simulink model "ML_2L_GFL_Y_Measure_AC_Sweep_2023"  (R2021b)
settings: Solver=ode23tb  StartTime=0.0  StopTime=1  FixedStep=Ts_Power  RelTol=1e-5
PreLoadFcn:
  | %Ts_Power=10e-6;
  | %Ts_Control=50e-6;
  | % System parameters
  | %Vl_l  = 400;   			        % Grid line-to-line voltage (Vrms)
  | %Vg_peak = Vl_l/sqrt(3)*sqrt(2); % Grid phase voltage (Vpk)
  | fg     = 50;	  			        % grid frequency (Hz)
  | %P = 30e3;
  | %Q = 0;
  | % LCL Filter parameters
  | L1=3e-3;
  | R_L1=80e-3;
  | L2=1.7e-3;
  | R_L2=22.3e-3;
  | C1=2e-6;
  | R_C1=7+21.5e-3;
  | % DC-link parameters
  | Vdc = 700;             	% DC voltage (V)
  | C=1500e-6;					% DC-link capacitance (F)
  | ESP=1e-3;
  | % Control parameters
  | fs = 10e3; 					% Switching frequency (Hz)
  | ts = 1/fs; 					% Switching period (s)
  | % Device parameters
  | Ron=1e-3;
  | 
  | 
  | 
  | % Circuit parameters
  | %Pr = 10000;            % Rated power (W)
  | %Zb = Vg_rms^2/Pr;     	% Base impedance (Ohm)
  | %Lg = 0.1*Zb/(2*pi*fac);% Grid connecting reactance (H)
  | %Rg = 0.01*Zb;         	% Grid connecting resistance (Ohm)
  | 
  | % Determining initial conditions
  | %Zinv = Rg + 1i*2*pi*fac*Lg;% Connecting impedance (Ohm,complex)
  | %Iref = Pr/(3*Vg_rms);      % Reference current (Irms)
  | %Vinv = Vg_rms + Iref*Zinv; % VSI generated voltage (Vrms,complex)
  | %Vinv_rms = abs(Vinv);      % VSI generated voltage magnitude (Vrms)
  | %Vinv_angle= angle(Vinv);   % VSI generated voltage angle (Rads)
  | 
  | %phase_balanced = 2*pi/3*[0 -1 1]; % Ideal balanced three-phase angles (Rads)
  | 
  | % Sine and Space Vector PWM parameters
  | %Vref = Vinv_rms*sqrt(2);  	% Reference voltage amplitude (V)
  | %phase_sine  = phase_balanced + Vinv_angle;   % Angles for sine PWM reference (Rads)
  | %phase_svpwm = phase_balanced + Vinv_angle ...% Angles for space vector PWM reference (Rads)
  | %                             + 2*pi*(fac/fs/2);
  | 
  | % Hystersis controller parameters
  | %Iout = Iref*sqrt(2);   			% Output current amplitude (A)
  | %Iband_hyst = Iout*0.2; 			% Hystersis current controller deadband (A)
  | %phase_hyst = phase_balanced; 	% Angles for hysteresis current reference (Rads)
  | 
  | % Remove complex variables from workspace
  | %clear('Zinv','Vinv')
InitFcn:
  | %Ts_Power=10e-6;
  | %Ts_Control=50e-6;
  | % System parameters
  | %Vl_l  = 400;   			        % Grid line-to-line voltage (Vrms)
  | %Vg_peak = Vl_l/sqrt(3)*sqrt(2); % Grid phase voltage (Vpk)
  | fg     = 50;	  			        % grid frequency (Hz)
  | %P = 30e3;
  | %Q = 0;
  | % LCL Filter parameters
  | L1=3e-3;
  | R_L1=80e-3;
  | L2=1.7e-3;
  | R_L2=22.3e-3;
  | C1=2e-6;
  | R_C1=7+21.5e-3;
  | % DC-link parameters
  | Vdc = 700;             	% DC voltage (V)
  | C=1500e-6;					% DC-link capacitance (F)
  | ESP=1e-3;
  | % Control parameters
  | fs = 10e3; 					% Switching frequency (Hz)
  | ts = 1/fs; 					% Switching period (s)
  | % Device parameters
  | Ron=1e-3;
  | 
  | 
  | 
  | % Circuit parameters
  | %Pr = 10000;            % Rated power (W)
  | %Zb = Vg_rms^2/Pr;     	% Base impedance (Ohm)
  | %Lg = 0.1*Zb/(2*pi*fac);% Grid connecting reactance (H)
  | %Rg = 0.01*Zb;         	% Grid connecting resistance (Ohm)
  | 
  | % Determining initial conditions
  | %Zinv = Rg + 1i*2*pi*fac*Lg;% Connecting impedance (Ohm,complex)
  | %Iref = Pr/(3*Vg_rms);      % Reference current (Irms)
  | %Vinv = Vg_rms + Iref*Zinv; % VSI generated voltage (Vrms,complex)
  | %Vinv_rms = abs(Vinv);      % VSI generated voltage magnitude (Vrms)
  | %Vinv_angle= angle(Vinv);   % VSI generated voltage angle (Rads)
  | 
  | %phase_balanced = 2*pi/3*[0 -1 1]; % Ideal balanced three-phase angles (Rads)
  | 
  | % Sine and Space Vector PWM parameters
  | %Vref = Vinv_rms*sqrt(2);  	% Reference voltage amplitude (V)
  | %phase_sine  = phase_balanced + Vinv_angle;   % Angles for sine PWM reference (Rads)
  | %phase_svpwm = phase_balanced + Vinv_angle ...% Angles for space vector PWM reference (Rads)
  | %                             + 2*pi*(fac/fs/2);
  | 
  | % Hystersis controller parameters
  | %Iout = Iref*sqrt(2);   			% Output current amplitude (A)
  | %Iband_hyst = Iout*0.2; 			% Hystersis current controller deadband (A)
  | %phase_hyst = phase_balanced; 	% Angles for hysteresis current reference (Rads)
  | 
  | % Remove complex variables from workspace
  | %clear('Zinv','Vinv')
StartFcn:
  | %Ts_Power=10e-6;
  | %Ts_Control=50e-6;
  | % System parameters
  | %Vl_l  = 400;   			        % Grid line-to-line voltage (Vrms)
  | %Vg_peak = Vl_l/sqrt(3)*sqrt(2); % Grid phase voltage (Vpk)
  | fg     = 50;	  			        % grid frequency (Hz)
  | %P = 30e3;
  | %Q = 0;
  | % LCL Filter parameters
  | L1=3e-3;
  | R_L1=80e-3;
  | L2=1.7e-3;
  | R_L2=22.3e-3;
  | C1=2e-6;
  | R_C1=7+21.5e-3;
  | % DC-link parameters
  | Vdc = 700;             	% DC voltage (V)
  | C=1500e-6;					% DC-link capacitance (F)
  | ESP=1e-3;
  | % Control parameters
  | fs = 10e3; 					% Switching frequency (Hz)
  | ts = 1/fs; 					% Switching period (s)
  | % Device parameters
  | Ron=1e-3;
  | 
  | 
  | 
  | % Circuit parameters
  | %Pr = 10000;            % Rated power (W)
  | %Zb = Vg_rms^2/Pr;     	% Base impedance (Ohm)
  | %Lg = 0.1*Zb/(2*pi*fac);% Grid connecting reactance (H)
  | %Rg = 0.01*Zb;         	% Grid connecting resistance (Ohm)
  | 
  | % Determining initial conditions
  | %Zinv = Rg + 1i*2*pi*fac*Lg;% Connecting impedance (Ohm,complex)
  | %Iref = Pr/(3*Vg_rms);      % Reference current (Irms)
  | %Vinv = Vg_rms + Iref*Zinv; % VSI generated voltage (Vrms,complex)
  | %Vinv_rms = abs(Vinv);      % VSI generated voltage magnitude (Vrms)
  | %Vinv_angle= angle(Vinv);   % VSI generated voltage angle (Rads)
  | 
  | %phase_balanced = 2*pi/3*[0 -1 1]; % Ideal balanced three-phase angles (Rads)
  | 
  | % Sine and Space Vector PWM parameters
  | %Vref = Vinv_rms*sqrt(2);  	% Reference voltage amplitude (V)
  | %phase_sine  = phase_balanced + Vinv_angle;   % Angles for sine PWM reference (Rads)
  | %phase_svpwm = phase_balanced + Vinv_angle ...% Angles for space vector PWM reference (Rads)
  | %                             + 2*pi*(fac/fs/2);
  | 
  | % Hystersis controller parameters
  | %Iout = Iref*sqrt(2);   			% Output current amplitude (A)
  | %Iband_hyst = Iout*0.2; 			% Hystersis current controller deadband (A)
  | %phase_hyst = phase_balanced; 	% Angles for hysteresis current reference (Rads)
  | 
  | % Remove complex variables from workspace
  | %clear('Zinv','Vinv')
undefined symbols (not defined in the file): fmax, fmin, plecs
libraries: plecslib_extras2 x1
settings Model: Creator=Lee  LastModifiedBy=DavinciL
settings SolverCC: AlgebraicLoopSolver=TrustRegion
settings DataIOCC: LimitDataPoints=on  SaveFormat=Array  ReturnWorkspaceOutputs=off
settings OptimizationCC: ExpressionDepthLimit=2147483647  EfficientMapNaN2IntZero=off  LifeSpan=inf
settings DebuggingCC: UnderspecifiedInitializationDetection=Classic  MergeDetectMultiDrivingBlocksExec=none  SolverPrmCheckMsg=warning  FcnCallInpInsideContextMsg=warning  UnconnectedInputMsg=none  UnconnectedOutputMsg=none  UnconnectedLineMsg=none  StateNameClashWarn=warning  SFUnexpectedBacktrackingDiag=warning  SFNoUnconditionalDefaultTransitionDiag=warning  SFExecutionAtInitializationDiag=none  SFMachineParentedDataDiag=warning  ArithmeticOperatorsInVariantConditions=warning
settings HardwareCC: ProdBitPerPointer=32  ProdBitPerSizeT=32  ProdBitPerPtrDiffT=32  ProdLargestAtomicFloat=None  ProdIntDivRoundTo=Undefined  ProdEndianess=Unspecified  ProdWordSize=32  ProdHWDeviceType=32-bit Generic  TargetBitPerPointer=64  TargetBitPerSizeT=64  TargetBitPerPtrDiffT=64  TargetLongLongMode=on  TargetIntDivRoundTo=Zero  TargetEndianess=LittleEndian  TargetWordSize=64  TargetHWDeviceType=MATLAB Host  ProdEqTarget=off
settings ModelReferenceCC: PropagateSignalLabelsOutOfModel=off
settings SFSimCC: SimUseLocalCustomCode=off  CustomCodeUndefinedFunction=UseInterfaceOnly
settings RTWCC: RTWUseLocalCustomCode=off
settings CodeAppCC: MaxIdLength=128  StateflowObjectComments=on
settings GRTTargetCC: TargetLangStandard=C89/C90 (ANSI)  CombineOutputUpdateFcns=off  GRTInterface=on
settings ConfigComp: CovMetricSettings=dw  CovSaveCumulativeToWorkspaceVar=on  CovSaveSingleToWorkspaceVar=on  CovExternalEMLEnable=off

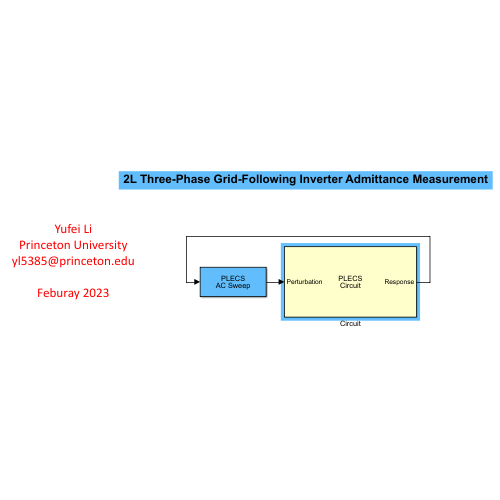
[thumbnail: Simulink's stored preview of the top-level diagram]
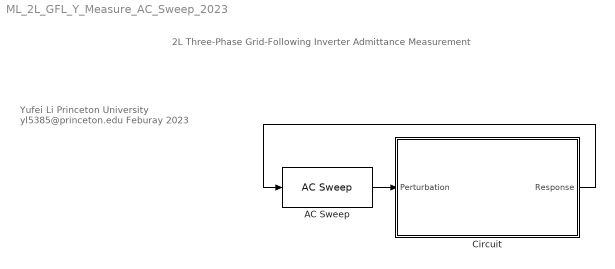
== system ML_2L_GFL_Y_Measure_AC_Sweep_2023 ==
  note: 2L Three-Phase Grid-Following Inverter Admittance Measurement
  note: Yufei Li
      | Princeton University
      | yl5385@princeton.edu
      |
      | Feburay 2023
  AC Sweep : plecslib_extras2/Analysis Tools/AC Sweep  FreqRange=[fmin fmax]  FreqScale=logarithmic  NPoints=N  InitialAmplitude=Vperturb  TimeSpan=1/50  TStart=0.1  ShowRefInput=off  Method=Steady-state analysis - start from unperturbed steady state  MaxIter=50  Tolerance=1e-4  Display=final  HideScopes=off  HiddenStates=error  OutputName=Y  BodePlot=off  JPert=1e-4  NInitCycles=0
      settings: SourceProductName=PLECS Extras
  Circuit : Subsystem  LoadFcn=plecs('sl', 200);  InitFcn=plecs('sl', 214);  StartFcn=plecs('sl', 208);  StopFcn=plecs('sl', 209);  mask(PlecsCircuit){PLECSData=<binary blob, 17988 chars, not shown>}
      mask prompts: PLECSData "PLECS Data (Do not delete or modify!)"
      mask init:
      | % PLACE CUSTOM INITIALIZATIONS ABOVE
      | % DO NOT REMOVE
      | plecs('sl', 215);
      | % DO NOT REMOVE
      settings: CopyFcn=plecs('sl', 203);  DeleteFcn=plecs('sl', 205);  UndoDeleteFcn=plecs('sl', 206);  PreSaveFcn=plecs('sl', 211);  PostSaveFcn=plecs('sl', 201);  NameChangeFcn=plecs('sl', 210);  DestroyFcn=plecs('sl', 207);  PreCopyFcn=plecs('sl', 216);  OpenFcn=plecs('sl', 202);  ErrorFcn=plerrorfcn
      mask Help: web(['file:///' fullfile(plecsdoc, 'creatingacircuit.html')])
      mask Display: disp('PLECS\nCircuit')
  wires:
  AC Sweep/1 -> Circuit/1(Perturbation)
  Circuit/1(Response) -> AC Sweep/1

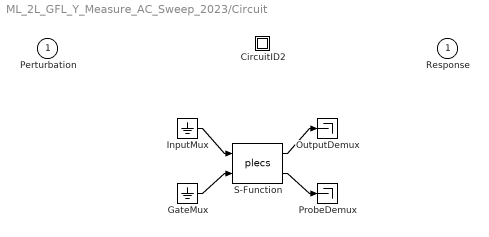
== system ML_2L_GFL_Y_Measure_AC_Sweep_2023/Circuit ==
  Perturbation : Inport  PortDimensions=1
  " CircuitID2 " : Subsystem
  " GateMux " : Ground
  " InputMux " : Ground
  " OutputDemux " : Terminator
  " ProbeDemux " : Terminator
  " S-Function " : S-Function  FunctionName=plecs  SFunctionDeploymentMode=off  EnableBusSupport=off
  Response : Outport  PortDimensions=1
  wires:
  " InputMux "/1 -> " S-Function "/1
  " GateMux "/1 -> " S-Function "/2
  " S-Function "/1 -> " OutputDemux "/1
  " S-Function "/2 -> " ProbeDemux "/1

== system ML_2L_GFL_Y_Measure_AC_Sweep_2023/Circuit/ CircuitID2  ==
